simulink model "simplificado"  (R2023a)
settings: Solver=VariableStepAuto  StartTime=0.0  StopTime=400  RelTol=1e-3
values from neighbouring files (symbols this model uses):
  A1 = 0.0154    [parametros.m]    (also in variables.mat)
  A2 = 5e-5    (= 5e-05)    [parametros.m]    (also in variables.mat)
  az = 0.5    [parametros.m]    (also in variables.mat)
  g = 9.8    [parametros.m]    (also in variables.mat)
  H_star = H_max/2    (= 0.31)    [parametros.m]    (also in variables.mat)
  Q_star = ro*A2*az*sqrt(2*g*H_star)    [parametros.m]    (also in variables.mat = 0.0616238590158)
  ro = 1000    [parametros.m]    (also in variables.mat)
libraries: fuzblock x1
settings Model: Creator=empg0  LastModifiedBy=empg0

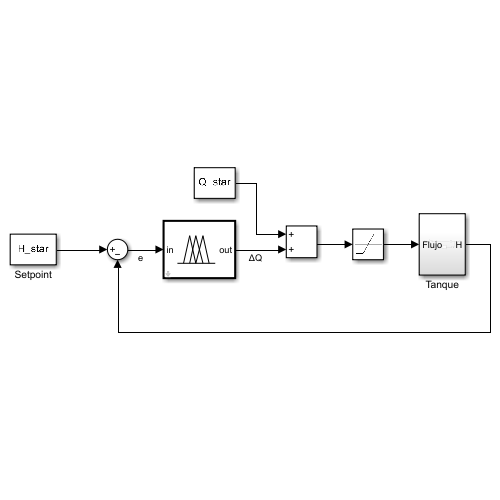
[thumbnail: Simulink's stored preview of the top-level diagram]
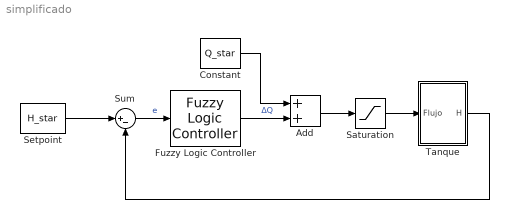
== system simplificado ==
  Add : Sum
  Constant : Constant  Value=Q_star
  Fuzzy Logic Controller : fuzblock/Fuzzy Logic  Controller  FIS='error_fuzzy.fis'  OutputSampleNumber=101  DataType=double  FuzzifiedInputs=off  RuleFiringStrengths=off  RuleOutputs=off  AggregatedOutputs=off  SimulateUsing=Interpreted execution  OutOfRangeInputValueMessage=warning  NoRuleFiredMessage=warning  EmptyOutputFuzzySetMessage=warning
  Saturation : Saturate  UpperLimit=0.1  LowerLimit=0
  Setpoint : Constant  Value=H_star
  Sum : Sum  Inputs=|+-
  Tanque : Subsystem
  wires:
  Constant/1 -> Add/1
  Tanque/1(H) -> Sum/2
  Sum/1 -> Fuzzy Logic Controller/1  "e"
  Fuzzy Logic Controller/1 -> Add/2  "ΔQ"
  Add/1 -> Saturation/1
  Saturation/1 -> Tanque/1(Flujo)
  Setpoint/1 -> Sum/1

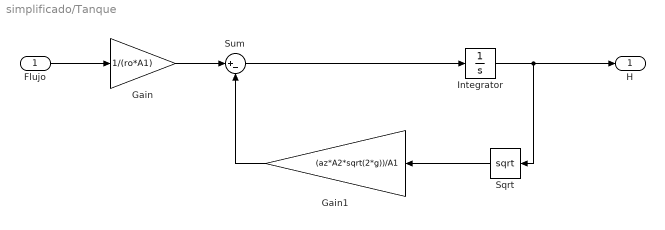
== system simplificado/Tanque ==
  Flujo : Inport
  Gain : Gain  Gain=1/(ro*A1)
  Gain1 : Gain  Gain=(az*A2*sqrt(2*g))/A1
  Integrator : Integrator  LimitOutput=on  UpperSaturationLimit=0.62  LowerSaturationLimit=0
  Sqrt : Sqrt
  Sum : Sum  Inputs=|+-
  H : Outport
  wires:
  Gain/1 -> Sum/1
  Sum/1 -> Integrator/1
  Sqrt/1 -> Gain1/1
  Gain1/1 -> Sum/2
  Integrator/1 -> H/1, Sqrt/1
  Flujo/1 -> Gain/1
